simulink model "thyristor_3phase_bridge"  (R2015a)
settings: Solver=ode45  StartTime=0.0  StopTime=0.09  MaxStep=1/1000  RelTol=1e-3
libraries: powerlib x14, simulink x6
settings Model: Creator=Windows 10  LastModifiedBy=Windows 10

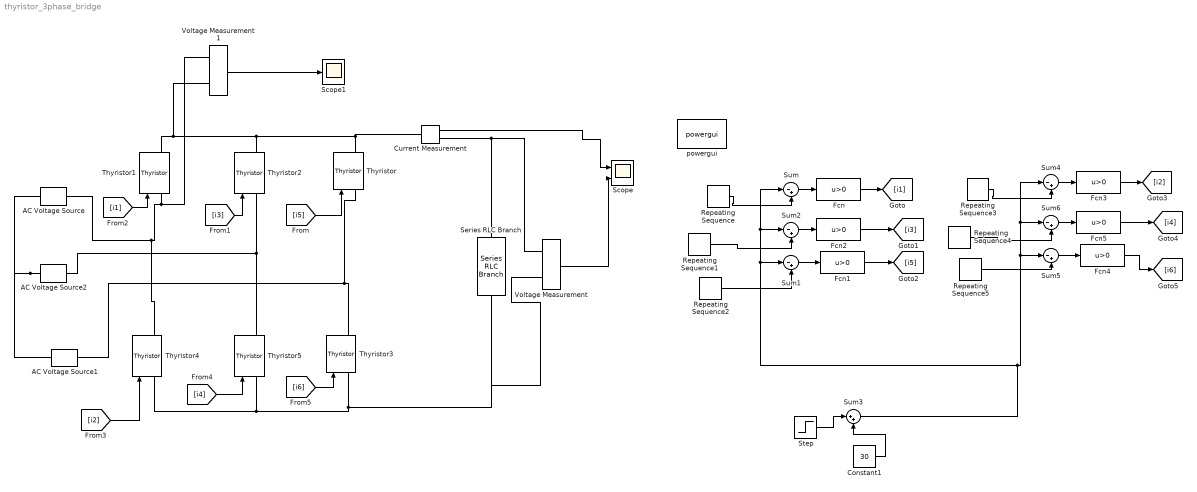
== system thyristor_3phase_bridge ==
  AC Voltage Source : powerlib/Electrical Sources/AC Voltage Source  Amplitude=300  Phase=0  Frequency=50  SampleTime=0  Measurements=None
  AC Voltage Source1 : powerlib/Electrical Sources/AC Voltage Source  Amplitude=300  Phase=120  Frequency=50  SampleTime=0  Measurements=None
  AC Voltage Source2 : powerlib/Electrical Sources/AC Voltage Source  Amplitude=300  Phase=-120  Frequency=50  SampleTime=0  Measurements=None
  Constant1 : Constant  Value=30
  Current Measurement : powerlib/Measurements/Current Measurement  PhasorSimulation=off  OutputType=Complex  PSBequivalent=0
  Fcn{,1..5} (6 alike) : Fcn  Expr=u>0
  Repeating Sequence : simulink/Sources/Repeating Sequence  rep_seq_t=[0 10 10.0001 20]*1e-3  rep_seq_y=[0 180 -180 0]
  Repeating Sequence1 : simulink/Sources/Repeating Sequence  rep_seq_t=[0 5*20/6 (5*20/6+0.0010) 20]*1e-3  rep_seq_y=[-120 180 -180 -120]
  Repeating Sequence2 : simulink/Sources/Repeating Sequence  rep_seq_t=[0 20/6 20/6+0.001 20]*1e-3  rep_seq_y=[120 180 -180 120]
  Repeating Sequence3 : simulink/Sources/Repeating Sequence  rep_seq_t=[0 20 20.0001]*1e-3  rep_seq_y=[-180 180 -180]
  Repeating Sequence4 : simulink/Sources/Repeating Sequence  rep_seq_t="[0  20/3  (20/3+0.0010) 20]*1e-3"  rep_seq_y=[60 180 -180 60]
  Repeating Sequence5 : simulink/Sources/Repeating Sequence  rep_seq_t=[0 40/3 40/3+0.001 20]*1e-3  rep_seq_y=[-60 180 -180 -60]
  Scope : Scope  NumInputPorts=2
      settings: YMin=-5~-5  YMax=5~5
  Scope1 : Scope
  Series RLC Branch : powerlib/Elements/Series RLC Branch  LConnTagsString=__new0  RConnTagsString=__new0  BranchType=RL  Resistance=2  Inductance=10e-3  SetiL0=off  InitialCurrent=0  Capacitance=1e-6  Setx0=off  InitialVoltage=0  Measurements=None
  Step : Step  Time=0.05  Before=30  After=60  SampleTime=0
  Sum{,1..2,4..6} (6 alike) : Sum  Inputs=|-+
  Sum3 : Sum  Inputs=|++
  Thyristor{,1..5} (6 alike) : powerlib/Power Electronics/Thyristor  Ron=0.001  Lon=0  Vf=0.8  IC=0  Rs=500  Cs=250e-9  Measurements=on
  Voltage Measurement : powerlib/Measurements/Voltage Measurement  PhasorSimulation=off  OutputType=Complex  PSBequivalent=0
  Voltage Measurement1 : powerlib/Measurements/Voltage Measurement  PhasorSimulation=off  OutputType=Complex  PSBequivalent=0
  powergui : powerlib/powergui  Priority=1  SimulationMode=Continuous  SolverType=Tustin/Backward Euler (TBE)  SampleTime=50e-6  frequency=60  SPID=off  DisableSnubberDevices=off  DisableRonSwitches=off  DisableVfSwitches=off  SwTol=0  DisplayEquations=off  Interpol=off  methode=off  Ts=100  FunctionMessages=off  echomessages=off  HookPort=off  EnableUseOfTLC=off  x0status=blocks  frequencyindice=50  Pbase=100e6  ErrMax=1e-4  Iterations=50  UnitsV=kV  UnitsW=MW  buscounter=0  RestoreLinks=warning  ResistiveCurrentMeasurement=off  Frange=[0:2:500]  Ylog=off  Xlog=on  ShowGrid=off  save=off  variable=ZData  structure=0  ZoomFFT=off  StartTime=0.0  cycles=1  DisplayStyle=1  fundamental=60  FreqAxis=off  MaxFrequency=1000  frequencyindicesteady=1  RmsSteady=1  display=off
  wires:
  Current Measurement/1 -> Scope/1
  Repeating Sequence/1 -> Sum/2
  Repeating Sequence1/1 -> Sum2/2
  Repeating Sequence2/1 -> Sum1/2
  Step/1 -> Sum3/1
  Constant1/1 -> Sum3/2
  Sum2/1 -> Fcn2/1
  Sum1/1 -> Fcn1/1
  Sum/1 -> Fcn/1
  Fcn2/1 -> [i3]
  Fcn1/1 -> [i5]
  Fcn/1 -> [i1]
  [i1] -> Thyristor1/1
  [i3] -> Thyristor2/1
  [i5] -> Thyristor/1
  [i2] -> Thyristor4/1
  [i4] -> Thyristor5/1
  [i6] -> Thyristor3/1
  Repeating Sequence3/1 -> Sum4/2
  Repeating Sequence4/1 -> Sum6/2
  Repeating Sequence5/1 -> Sum5/2
  Sum3/1 -> Sum1/1, Sum2/1, Sum/1, Sum5/1, Sum6/1, Sum4/1
  Sum6/1 -> Fcn5/1
  Sum5/1 -> Fcn4/1
  Sum4/1 -> Fcn3/1
  Fcn5/1 -> [i4]
  Fcn4/1 -> [i6]
  Fcn3/1 -> [i2]
  Voltage Measurement/1 -> Scope/2
  Voltage Measurement1/1 -> Scope1/1
  connections:
  AC Voltage Source2/LConn1 -- AC Voltage Source1/LConn1 -- AC Voltage Source/LConn1
  Series RLC Branch/LConn1 -- Current Measurement/RConn1 -- Voltage Measurement/LConn1
  Thyristor1/LConn1 -- AC Voltage Source/RConn1 -- Thyristor4/RConn1 -- Voltage Measurement1/LConn1
  Thyristor2/LConn1 -- Thyristor5/RConn1 -- AC Voltage Source2/RConn1
  Thyristor/LConn1 -- AC Voltage Source1/RConn1 -- Thyristor3/RConn1
  Thyristor4/LConn1 -- Series RLC Branch/RConn1 -- Voltage Measurement/LConn2 -- Thyristor3/LConn1 -- Thyristor5/LConn1
  Thyristor1/RConn1 -- Thyristor/RConn1 -- Current Measurement/LConn1 -- Thyristor2/RConn1 -- Voltage Measurement1/LConn2
